simulink model "motor_model"  (R2023b)
settings: Solver=VariableStepAuto  StartTime=0.0  StopTime=24  RelTol=1e-3
libraries: simulink x1
settings Model: Creator=user  LastModifiedBy=user

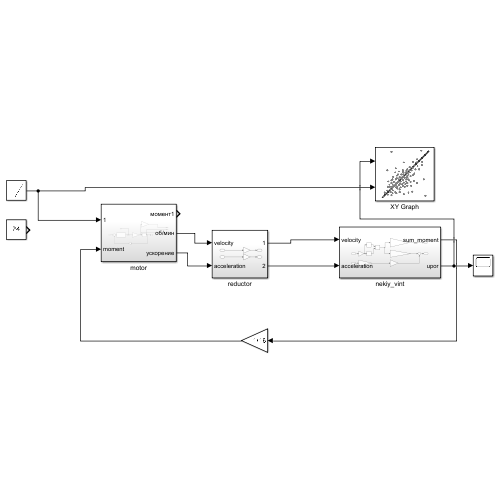
[thumbnail: Simulink's stored preview of the top-level diagram]
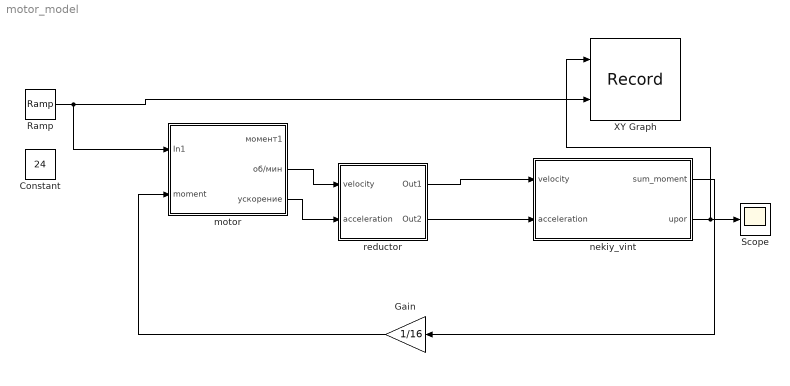
== system motor_model ==
  Constant : Constant  Value=24
  Gain : Gain  Gain=1/16
  Ramp : simulink/Sources/Ramp  slope=2  start=0  InitialOutput=-24
  Scope : Scope
  XY Graph : Record  FileSettingsInternal="{\"entries\":[{\"content\":{\"excelSettings\":{\"content\":{},\"type\":\"Streamout.ExcelSettings\"}},\"type\":\"Streamout.FileSettingStorage\",\"uuid\":\"\"}],\"packageUris\":[\"http:\\/\\/schema.mathworks.com\\/mf0\\/streamout_blocks\\/R2020a\"],\"version\":\"1.0\"}"  Layout=[1 1]  SignalsInternal="{\"entries\":[{\"content\":{\"signals\":[{\"content\":{\"blockPath\":[],\"dimensions\":[1],\"domain\":\"\",\"lineColor\":\"#edb120\",\"plots\":[1],\"port\":1,\"sid\":[\"\"],\"signalID\":330,\"signalName\":\"nekiy_vint:2\"},\"type\":\"RecordBlkView.Signal\",\"uuid\":\"\"},{\"content\":{\"blockPath\":[],\"dimensions\":[1],\"domain\":\"\",\"lineColor\":\"#7e2f8e\",\"plots\":[1],\"port\":2,\"sid\":[\"\"],\"signalID\":334,\"signalName\":\"Ramp\"},\"type\":\"RecordBlkView.Signal\",\"uuid\":\"\"}]},\"type\":\"RecordBlkView.InputSignals\",\"uuid\":\"\"}],\"packageUris\":[\"http:\\/\\/schema.mathworks.com\\/mf0\\/streamout_blocks\\/R2020a\"],\"version\":\"1.0\"}"  VisualizationBindings="{\"xyplotplugin\":{\"info\":[{\"series\":[{\"bindingParametersList\":[{\"parameter\":\"X-Axis\",\"signalID\":334,\"signalName\":\"Ramp\"},{\"parameter\":\"Y-Axis\",\"signalID\":330,\"signalName\":\"nekiy_vint:2\"}],\"seriesID\":54987}],\"subplotID\":1}]}}"  CompatibilityTag=XY
  motor : Subsystem
  nekiy_vint : Subsystem
  reductor : Subsystem
  wires:
  motor/3(ускорение) -> reductor/2(acceleration)
  motor/2(об/мин) -> reductor/1(velocity)
  reductor/1(Out1) -> nekiy_vint/1(velocity)
  reductor/2(Out2) -> nekiy_vint/2(acceleration)
  nekiy_vint/1(sum_moment) -> Gain/1
  nekiy_vint/2(upor) -> XY Graph/1, Scope/1
  Gain/1 -> motor/2(moment)
  Ramp/1 -> motor/1(In1), XY Graph/2

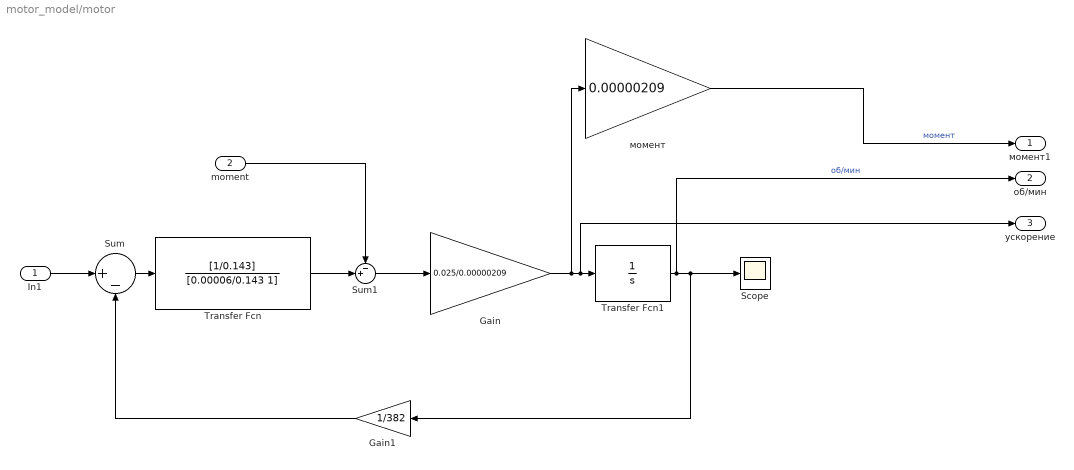
== system motor_model/motor ==
  In1 : Inport
  moment : Inport  Port=2
  Gain : Gain  Gain=0.025/0.00000209
  Gain1 : Gain  Gain=1/382
  Scope : Scope
  Sum : Sum  Inputs=|+-
  Sum1 : Sum  Inputs=-+|
  Transfer Fcn : TransferFcn  Numerator=[1/0.143]  Denominator=[0.00006/0.143 1]
  Transfer Fcn1 : TransferFcn  Denominator=[1 0]
  момент : Gain  Gain=0.00000209
  момент1 : Outport
  об/мин : Outport  Port=2
  ускорение : Outport  Port=3
  wires:
  Sum/1 -> Transfer Fcn/1
  Gain/1 -> ускорение/1, Transfer Fcn1/1, момент/1
  Transfer Fcn1/1 -> об/мин/1, Gain1/1, Scope/1  "об/мин"
  момент/1 -> момент1/1  "момент"
  Gain1/1 -> Sum/2
  In1/1 -> Sum/1
  Transfer Fcn/1 -> Sum1/2
  Sum1/1 -> Gain/1
  moment/1 -> Sum1/1

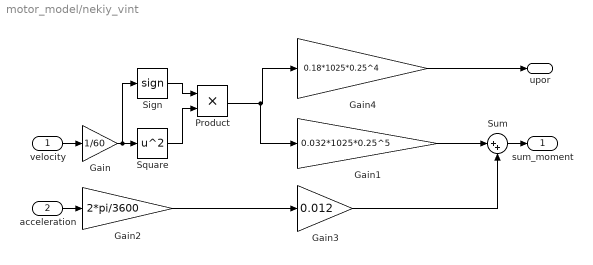
== system motor_model/nekiy_vint ==
  velocity : Inport
  acceleration : Inport  Port=2
  Gain : Gain  Gain=1/60
  Gain1 : Gain  Gain=0.032*1025*0.25^5
  Gain2 : Gain  Gain=2*pi/3600
  Gain3 : Gain  Gain=0.012
  Gain4 : Gain  Gain=0.18*1025*0.25^4
  Product : Product
  Sign : Signum
  Square : Math  Operator=square
  Sum : Sum  Inputs=|++
  sum_moment : Outport
  upor : Outport  Port=2
  wires:
  acceleration/1 -> Gain2/1
  Gain3/1 -> Sum/2
  velocity/1 -> Gain/1
  Sum/1 -> sum_moment/1
  Gain1/1 -> Sum/1
  Gain/1 -> Sign/1, Square/1
  Gain2/1 -> Gain3/1
  Gain4/1 -> upor/1
  Square/1 -> Product/2
  Sign/1 -> Product/1
  Product/1 -> Gain1/1, Gain4/1

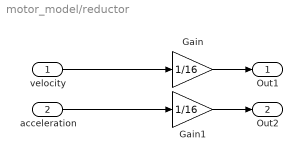
== system motor_model/reductor ==
  velocity : Inport
  acceleration : Inport  Port=2
  Gain : Gain  Gain=1/16
  Gain1 : Gain  Gain=1/16
  Out1 : Outport
  Out2 : Outport  Port=2
  wires:
  Gain1/1 -> Out2/1
  velocity/1 -> Gain/1
  acceleration/1 -> Gain1/1
  Gain/1 -> Out1/1
